simulink model "f16_simulink"  (R2021a)
settings: Solver=VariableStepAuto  StartTime=0.0  StopTime=30  FixedStep=0.01  MaxStep=0.1  RelTol=1e-3
values from neighbouring files (symbols this model uses):
  alpha_vec = -10:5:45    [f16_aeroFM.m]    (also in f16_controlFM.m; f16_simulink_setup.m)
  altitude_vec = 0:10000:50000    [f16_simulink_setup.m]    (also in f16_thrust.m)
  beta_vec10 = -30:10:30    [f16_controlFM.m]    (also in f16_simulink_setup.m)
  beta_vec5 = 0:5:30    [f16_aeroFM.m]    (also in f16_simulink_setup.m)
  Cz_lookup = [.770, .241, -.100, -.416, -.731, -1.053, -1.366, -1.646, -1.917, -2.120, -2.248, -2.229]    [f16_aeroFM.m]    (also in f16_simulink_setup.m)
  damp_table = [-.267, -.110, .308, 1.34, 2.08, 2.91, 2.76, 2.05, 1.50, 1.49, 1.83, 1.21 ... (first row only)    [f16_simulink_setup.m]
  elev_vec = -24:12:24    [f16_aeroFM.m]    (also in f16_simulink_setup.m)
  GAM = mass.Jxx*mass.Jzz - mass.Jxz^2    [f16_dynamics.m]    (also in f16_simulink_setup.m)
  Kp = 0.65    [f16_simulink_DAQ.m]
  Kpi = 0.01    [f16_simulink_DAQ.m]
  Kt = 0.439    [f16_simulink_DAQ.m]
  Mach_vec = linspace(0,1,6)    [f16_simulink_setup.m]    (also in f16_thrust.m)
  OL_cmd = 15    [f16_simulink_DAQ.m]
  pilot_delay = 0.15    [f16_simulink_DAQ.m]
  pitch_limiter = 70    [f16_simulink_DAQ.m]
  pow_vec = [0 50 100]    [f16_simulink_setup.m]    (also in f16_thrust.m)
  power_table = cat(3,throt1',throt2',throt3')    [f16_simulink_setup.m]
  pulse_on = 0    [f16_simulink_DAQ.m]
  r2d = 57.29578    [f16_dynamics.m]    (also in f16_simulink_setup.m = 57.2957795131)
  ratelim_on = 1    [f16_simulink_DAQ.m]
  rho0 = 2.377e-3    (= 0.002377)    [f16_simulink_setup.m]
  thetaref_amp = 20    [f16_simulink_DAQ.m]
  thetaref_per = 4    [f16_simulink_DAQ.m]
  utrim = [smin(1) smin(2) smin(4) smin(5)]'    [f16_DAQ.m]    (also in f16_simulink_DAQ.m)
  wavestart = 5    [f16_simulink_DAQ.m]    (also in f16_simulink_setup.m)
  xcgr = 0.3    [f16_simulink_DAQ.m]
  xPQ = mass.Jxz*(mass.Jxx - mass.Jyy + mass.Jzz)    [f16_dynamics.m]    (also in f16_simulink_setup.m)
  xQR = mass.Jzz*(mass.Jzz-mass.Jyy) + mass.Jxz*2    [f16_dynamics.m]    (also in f16_simulink_setup.m)
  xtrim = x    [f16_DAQ.m]    (also in f16_simulink_DAQ.m)
  yPR = mass.Jzz - mass.Jxx    [f16_dynamics.m]    (also in f16_simulink_setup.m)
  zPQ = (mass.Jxx - mass.Jyy)*mass.Jxx + mass.Jxz^2    [f16_dynamics.m]    (also in f16_simulink_setup.m)
undefined symbols (not defined in the file or in its folder): ctrl, dims, mass
settings Model: Creator=loren  LastModifiedBy=loren

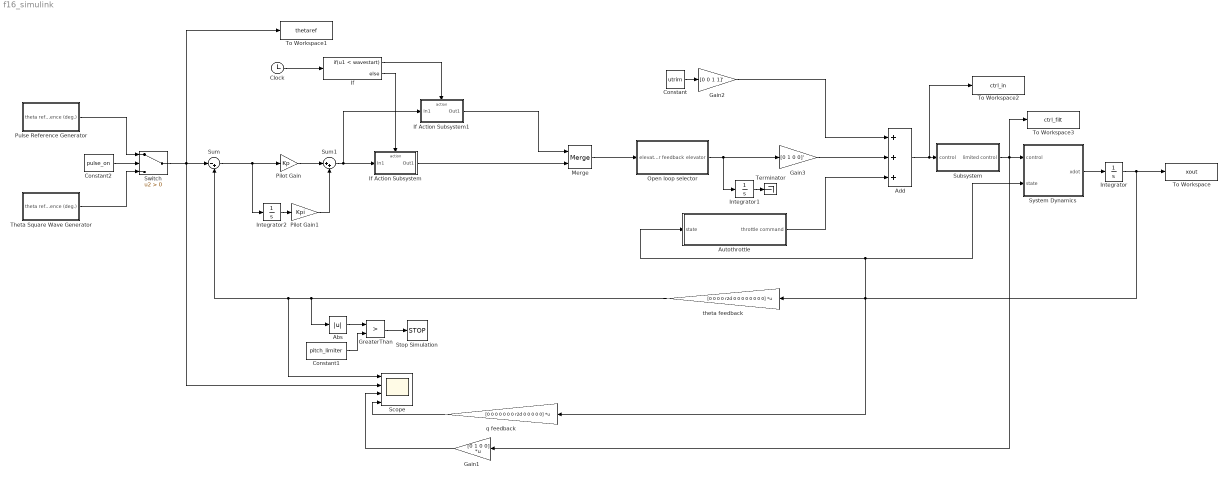
== system f16_simulink ==
  Abs : Abs
  Add : Sum  Inputs=+++
  Autothrottle : Subsystem
  Clock : Clock
  Constant : Constant  Value=utrim
  Constant1 : Constant  Value=pitch_limiter
  Constant2 : Constant  Value=pulse_on
  Gain1 : Gain  Gain=[0 1 0 0]  Multiplication=Matrix(K*u)
  Gain2 : Gain  Gain=[0 0 1 1]'
  Gain3 : Gain  Gain=[0 1 0 0]'
  GreaterThan : RelationalOperator  Operator=>  OutDataTypeStr=boolean  RndMeth=Simplest
  If : If  IfExpression=u1 < wavestart
  If Action Subsystem : Subsystem  TreatAsAtomicUnit=on
  If Action Subsystem1 : Subsystem  TreatAsAtomicUnit=on
  Integrator : Integrator  InitialCondition=xtrim
  Integrator1 : Integrator  InitialCondition=utrim(2)
  Integrator2 : Integrator  InitialCondition=utrim(2)*1000
  Merge : Merge
  Open loop selector : Subsystem
  Pilot Gain : Gain  Gain=Kp
  Pilot Gain1 : Gain  Gain=Kpi
  Pulse Reference Generator : Subsystem
  Scope : Scope  NumInputPorts=4
  Stop Simulation : Stop
  Subsystem : Subsystem
  Sum : Sum  Inputs=|-+
  Sum1 : Sum  Inputs=|++
  Switch : Switch  Criteria=u2 > Threshold
  System Dynamics : Subsystem
  Terminator : Terminator
  Theta Square Wave Generator : Subsystem
  To Workspace : ToWorkspace  VariableName=xout  SampleTime=-1
  To Workspace1 : ToWorkspace  VariableName=thetaref  SampleTime=-1
  To Workspace2 : ToWorkspace  VariableName=ctrl_in  SampleTime=-1
  To Workspace3 : ToWorkspace  VariableName=ctrl_filt  SampleTime=-1
  q feedback : Gain  Gain=[0 0 0 0 0 0 0 r2d 0 0 0 0 0]  Multiplication=Matrix(K*u)
  theta feedback : Gain  Gain=[0 0 0 0 r2d 0 0 0 0 0 0 0 0]  Multiplication=Matrix(K*u)
  wires:
  System Dynamics/1(xdot) -> Integrator/1
  Integrator/1 -> q feedback/1, theta feedback/1, Autothrottle/1(state), System Dynamics/2(state), To Workspace/1
  Switch/1 -> To Workspace1/1, Sum/1, Scope/2
  Sum1/1 -> If Action Subsystem1/1(In1), If Action Subsystem/1(In1)
  Subsystem/1(limited control) -> To Workspace3/1, Gain1/1, System Dynamics/1(control)
  Sum/1 -> Integrator2/1, Pilot Gain/1
  Add/1 -> To Workspace2/1, Subsystem/1(control)
  Constant/1 -> Gain2/1
  Gain2/1 -> Add/1
  Autothrottle/1(throttle command) -> Add/3
  theta feedback/1 -> Abs/1, Sum/2, Scope/1
  Gain1/1 -> Scope/3
  GreaterThan/1 -> Stop Simulation/1
  Abs/1 -> GreaterThan/1
  Constant1/1 -> GreaterThan/2
  Constant2/1 -> Switch/2
  Pulse Reference Generator/1(theta reference (deg.)) -> Switch/1
  Theta Square Wave Generator/1(theta reference (deg.)) -> Switch/3
  q feedback/1 -> Scope/4
  Gain3/1 -> Add/2
  Open loop selector/1(elevator) -> Integrator1/1, Gain3/1
  Integrator1/1 -> Terminator/1
  Integrator2/1 -> Pilot Gain1/1
  Pilot Gain1/1 -> Sum1/2
  Merge/1 -> Open loop selector/1(elevator feedback)
  Pilot Gain/1 -> Sum1/1
  Clock/1 -> If/1
  If Action Subsystem1/1(Out1) -> Merge/1
  If/2 -> If Action Subsystem/Action
  If/1 -> If Action Subsystem1/Action
  If Action Subsystem/1(Out1) -> Merge/2

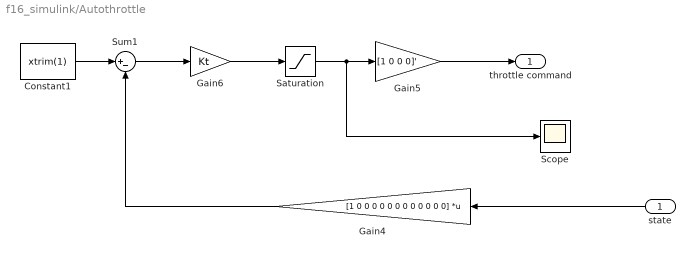
== system f16_simulink/Autothrottle ==
  state : Inport
  Constant1 : Constant  Value=xtrim(1)
  Gain4 : Gain  Gain=[1 0 0 0 0 0 0 0 0 0 0 0 0]  Multiplication=Matrix(K*u)
  Gain5 : Gain  Gain=[1 0 0 0]'
  Gain6 : Gain  Gain=Kt
  Saturation : Saturate  UpperLimit=1  LowerLimit=0.1
  Scope : Scope
  Sum1 : Sum  Inputs=|+-
  throttle command : Outport
  wires:
  Saturation/1 -> Scope/1, Gain5/1
  Sum1/1 -> Gain6/1
  Gain4/1 -> Sum1/2
  Gain5/1 -> throttle command/1
  state/1 -> Gain4/1
  Constant1/1 -> Sum1/1
  Gain6/1 -> Saturation/1

== system f16_simulink/If Action Subsystem ==
  In1 : Inport
  Action Port : ActionPort  ActionPortLabel=else
  Pilot Delay1 : TransportDelay  DelayTime=pilot_delay
  Out1 : Outport
  wires:
  In1/1 -> Pilot Delay1/1
  Pilot Delay1/1 -> Out1/1

== system f16_simulink/If Action Subsystem1 ==
  In1 : Inport
  Action Port : ActionPort  ActionPortLabel=if(u1 < wavestart)
  Out1 : Outport
  wires:
  In1/1 -> Out1/1

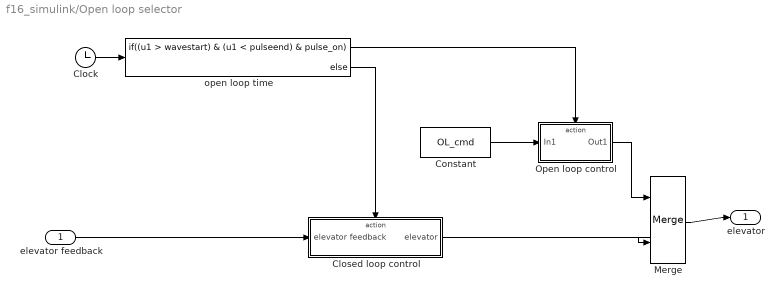
== system f16_simulink/Open loop selector ==
  elevator feedback : Inport
  Clock : Clock
  Closed loop control : Subsystem  TreatAsAtomicUnit=on
  Constant : Constant  Value=OL_cmd
  Merge : Merge
  Open loop control : Subsystem  TreatAsAtomicUnit=on
  open loop time : If  IfExpression=(u1 > wavestart) & (u1 < pulseend) & pulse_on
  elevator : Outport
  wires:
  Clock/1 -> open loop time/1
  Merge/1 -> elevator/1
  elevator feedback/1 -> Closed loop control/1(elevator feedback)
  open loop time/2 -> Closed loop control/Action
  Closed loop control/1(elevator) -> Merge/2
  Open loop control/1(Out1) -> Merge/1
  open loop time/1 -> Open loop control/Action
  Constant/1 -> Open loop control/1(In1)

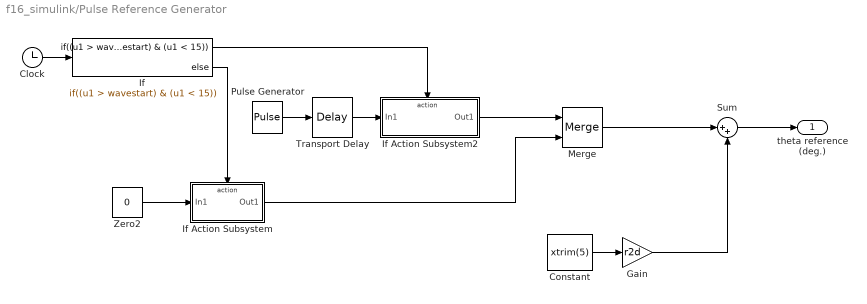
== system f16_simulink/Pulse Reference Generator ==
  Clock : Clock
  Constant : Constant  Value=xtrim(5)
  Gain : Gain  Gain=r2d
  If : If  IfExpression=(u1 > wavestart) & (u1 < 15)
  If Action Subsystem : Subsystem  TreatAsAtomicUnit=on
  If Action Subsystem2 : Subsystem  TreatAsAtomicUnit=on
  Merge : Merge
  Pulse Generator : DiscretePulseGenerator  PulseType=Time based  Amplitude=0  Period=20  PulseWidth=50
  Sum : Sum  Inputs=|++
  Transport Delay : TransportDelay  DelayTime=wavestart
  Zero2 : Constant  Value=0  OutDataTypeStr=Inherit: Inherit via back propagation
  theta reference (deg.) : Outport
  wires:
  Sum/1 -> theta reference (deg.)/1
  Pulse Generator/1 -> Transport Delay/1
  Gain/1 -> Sum/2
  Constant/1 -> Gain/1
  Merge/1 -> Sum/1
  If Action Subsystem2/1(Out1) -> Merge/1
  If/1 -> If Action Subsystem2/Action
  Clock/1 -> If/1
  If/2 -> If Action Subsystem/Action
  Transport Delay/1 -> If Action Subsystem2/1(In1)
  If Action Subsystem/1(Out1) -> Merge/2
  Zero2/1 -> If Action Subsystem/1(In1)

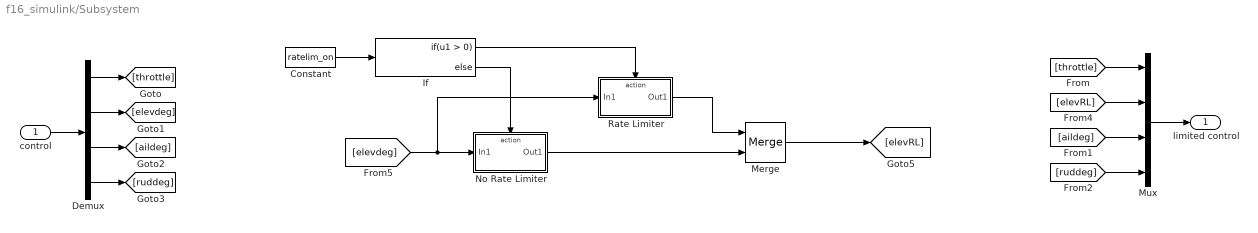
== system f16_simulink/Subsystem ==
  control : Inport
  Constant : Constant  Value=ratelim_on
  Demux : Demux
  If : If
  Merge : Merge
  Mux : Mux
  No Rate Limiter : Subsystem  TreatAsAtomicUnit=on
  Rate Limiter : Subsystem  TreatAsAtomicUnit=on
  limited control : Outport
  wires:
  Mux/1 -> limited control/1
  control/1 -> Demux/1
  Demux/1 -> [throttle]
  Demux/4 -> [ruddeg]
  Demux/3 -> [aildeg]
  Demux/2 -> [elevdeg]
  [throttle] -> Mux/1
  [aildeg] -> Mux/3
  [ruddeg] -> Mux/4
  [elevRL] -> Mux/2
  Constant/1 -> If/1
  If/2 -> No Rate Limiter/Action
  If/1 -> Rate Limiter/Action
  [elevdeg] -> Rate Limiter/1(In1), No Rate Limiter/1(In1)
  Rate Limiter/1(Out1) -> Merge/1
  Merge/1 -> [elevRL]
  No Rate Limiter/1(Out1) -> Merge/2

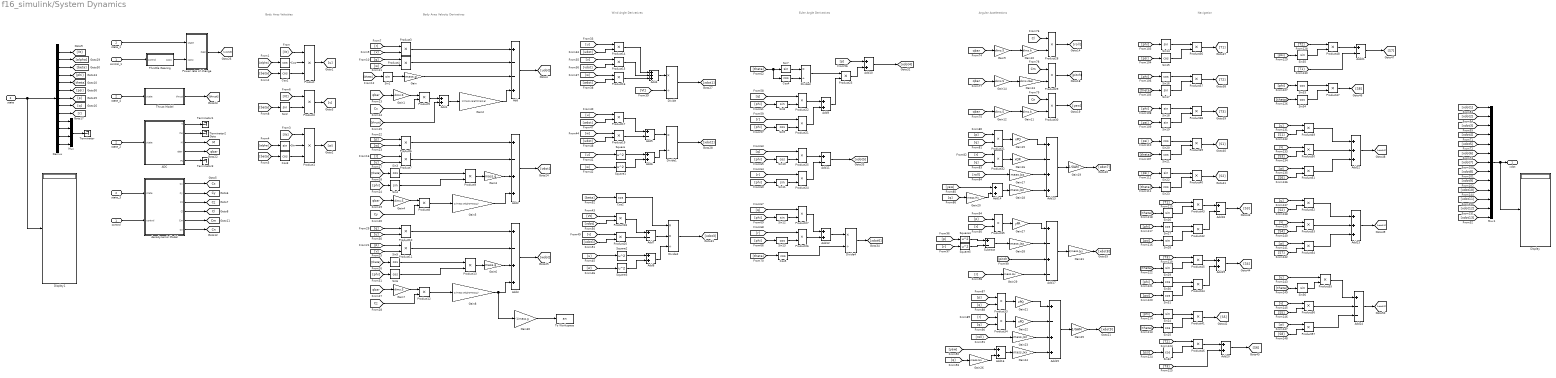
== system f16_simulink/System Dynamics ==
  note: Body Axes Velocities
  note: Body Axes Velocity Derivatives
  note: Wind Angle Derivatives
  note: Euler Angle Derivatives
  note: Angular Accelerations
  note: Navigation
  control : Inport
  state : Inport  Port=2
  ADC : Subsystem
  Add : Sum  Inputs=+--+
  Add{1,6,8..10,12,14,16,19..20} (10 alike) : Sum
  Add{5,7,11,18,21} (5 alike) : Sum  Inputs=+-
  Add{2..3,13,15} (4 alike) : Sum  Inputs=+-++
  Add17 : Sum  Inputs=+-+-
  Add22 : Sum  Inputs=+++
  Add23 : Sum  Inputs=+++
  Add24 : Sum  Inputs=+--
  Add4 : Sum  Inputs=+++
  Aerodynamic Model : Subsystem
  Cos{,1..5} (6 alike) : Trigonometry  Operator=cos
  Demux : Demux  Outputs=13
  Display : Display
  Display1 : Display
  Divide{,1,3..4} (4 alike) : Product  Inputs=*/
  Divide2 : Product  Inputs=**/
  Gain : Gain  Gain=mass.g
  Gain{1,4,7,9,12,14} (6 alike) : Gain  Gain=dims.S
  Gain10 : Gain  Gain=dims.b
  Gain11 : Gain  Gain=dims.b
  Gain13 : Gain  Gain=dims.cbar
  Gain15 : Gain  Gain=xPQ
  Gain16 : Gain  Gain=xQR
  Gain17 : Gain  Gain=mass.Jzz
  Gain18 : Gain  Gain=mass.Jxz
  Gain19 : Gain  Gain=1/GAM
  Gain2 : Gain  Gain=1/(mass.weight/mass.g)
  Gain20 : Gain  Gain=mass.Hx
  Gain21 : Gain  Gain=zPQ
  Gain22 : Gain  Gain=xPQ
  Gain23 : Gain  Gain=mass.Jxz
  Gain24 : Gain  Gain=mass.Jxx
  Gain25 : Gain  Gain=1/GAM
  Gain26 : Gain  Gain=mass.Hx
  Gain27 : Gain  Gain=yPR
  Gain28 : Gain  Gain=mass.Jxz
  Gain29 : Gain  Gain=mass.Hx
  Gain3 : Gain  Gain=mass.g
  Gain30 : Gain  Gain=-1/mass.g
  Gain31 : Gain  Gain=1/mass.Jyy
  Gain5 : Gain  Gain=1/(mass.weight/mass.g)
  Gain6 : Gain  Gain=mass.g
  Gain8 : Gain  Gain=1/(mass.weight/mass.g)
  Mux : Mux
  Mux1 : Mux  Inputs=13
  Power rate of change : Subsystem
  Product : Product  Inputs=3
  Product1 : Product  Inputs=3
  Product{2..57} (56 alike) : Product
  Sin{,1..2,4,7..8,11..12,14,17..19,22,24,26,28..29,35..36} (19 alike) : Trigonometry
  Sin{3,5..6,9..10,13,15..16,20..21,23,25,27,30..34} (18 alike) : Trigonometry  Operator=cos
  Square{,1..5} (6 alike) : Math  Operator=square  SaturateOnIntegerOverflow=on
  Subtract : Sum  Inputs=+-
  Terminator{,1..3} (4 alike) : Terminator
  Throttle Gearing : Subsystem
  Thrust Model : Subsystem
  To Workspace : ToWorkspace  VariableName=an  SampleTime=-1
  control_1 : InportShadow
  state_{1..4} (4 alike) : InportShadow  Port=2
  xdot : Outport
  tag scope: Cl=global, Cm=global, Cn=global, Cx=global, Cy=global, Cz=global, M=global, qbar=global
  wires:
  state_3/1 -> Aerodynamic Model/1(state)
  Add/1 -> [udot]
  [v] -> Product3/2
  [qbar] -> Gain1/1
  ADC/4(qbar) -> [qbar]
  Aerodynamic Model/1(Cx) -> [Cx]
  Thrust Model/1(thrust) -> [thrust]
  Gain/1 -> Add/3
  Mux1/1 -> Display/1, xdot/1
  Throttle Gearing/1(cpow) -> Power rate of change/2(cpow)
  [Vt] -> Product2/1
  [beta] -> Cos1/1
  Add1/1 -> Gain2/1
  ADC/3(M) -> [M]
  state/1 -> Display1/1, Demux/1
  [theta] -> Sin1/1
  Demux/1 -> [Vt]
  Aerodynamic Model/4(Cl) -> [Cl]
  control/1 -> Aerodynamic Model/2(control)
  Demux/13 -> Mux/4
  Demux/5 -> [theta]
  Demux/4 -> [phi]
  Product1/1 -> [w]
  Product2/1 -> [v]
  [Cx] -> Product5/2
  control_1/1 -> Throttle Gearing/1(control)
  state_2/1 -> ADC/1(state)
  Aerodynamic Model/3(Cz) -> [Cz]
  Gain1/1 -> Product5/1
  state_1/1 -> Power rate of change/1(state)
  [alpha] -> Cos/1
  Demux/11 -> Mux/2
  ADC/2(rho) -> Terminator2/1
  Demux/12 -> Mux/3
  Demux/9 -> [r]
  state_4/1 -> Thrust Model/1(state)
  Aerodynamic Model/5(Cm) -> [Cm]
  Aerodynamic Model/6(Cn) -> [Cn]
  [q] -> Product4/1
  [beta] -> Cos3/1
  Demux/7 -> [p]
  Demux/3 -> [beta]
  Aerodynamic Model/2(Cy) -> [Cy]
  Sin2/1 -> Product2/2
  [beta] -> Sin2/1
  Demux/2 -> [alpha]
  ADC/5(Ps) -> Terminator3/1
  Sin1/1 -> Gain/1
  Demux/8 -> [q]
  Mux/1 -> Terminator/1
  Product5/1 -> Add1/1
  Demux/6 -> [psi]
  Demux/10 -> Mux/1
  [Vt] -> Product1/1
  Sin/1 -> Product1/2
  Product3/1 -> Add/1
  [thrust] -> Add1/2
  Product/1 -> [u]
  Cos3/1 -> Product1/3
  [alpha] -> Sin/1
  Cos/1 -> Product/2
  [r] -> Product3/1
  Product4/1 -> Add/2
  [Vt] -> Product/1
  [w] -> Product4/2
  Cos1/1 -> Product/3
  Gain2/1 -> Add/4
  ADC/1(T) -> Terminator1/1
  Power rate of change/1(Pdot) -> [xdot13]
  Gain4/1 -> Product8/1
  [Cy] -> Product8/2
  [theta] -> Sin3/1
  Product8/1 -> Gain5/1
  [qbar] -> Gain4/1
  Sin3/1 -> Product9/1
  [w] -> Product6/2
  Add2/1 -> [vdot]
  Gain5/1 -> Add2/4
  [u] -> Product7/2
  Product7/1 -> Add2/2
  [p] -> Product6/1
  [r] -> Product7/1
  Product6/1 -> Add2/1
  Product9/1 -> Gain3/1
  [phi] -> Sin4/1
  Sin4/1 -> Product9/2
  Gain3/1 -> Add2/3
  [phi] -> Sin6/1
  [p] -> Product11/1
  [q] -> Product10/1
  Product11/1 -> Add3/2
  [Cz] -> Product12/2
  [u] -> Product10/2
  [qbar] -> Gain7/1
  [theta] -> Sin5/1
  Gain7/1 -> Product12/1
  Product12/1 -> Gain8/1
  Product10/1 -> Add3/1
  Add3/1 -> [wdot]
  Gain6/1 -> Add3/3
  Sin6/1 -> Product13/2
  Product13/1 -> Gain6/1
  Gain8/1 -> Gain30/1, Add3/4
  Sin5/1 -> Product13/1
  [v] -> Product11/2
  [xdot13] -> Mux1/13
  [u] -> Product14/1
  [udot] -> Product14/2
  [v] -> Product15/1
  [w] -> Product16/1
  [vdot] -> Product15/2
  [wdot] -> Product16/2
  Product15/1 -> Add4/2
  Product14/1 -> Add4/1
  Product16/1 -> Add4/3
  Add4/1 -> Divide/1
  [Vt] -> Divide/2
  Divide/1 -> [xdot1]
  [udot] -> Product19/2
  [wdot] -> Product17/2
  [u] -> Product17/1
  [w] -> Product19/1
  Product17/1 -> Add5/1
  Add5/1 -> Divide1/1
  Add6/1 -> Divide1/2
  Divide1/1 -> [xdot2]
  Product19/1 -> Add5/2
  [w] -> Square1/1
  Square1/1 -> Add6/2
  Square/1 -> Add6/1
  [u] -> Square/1
  [w] -> Square3/1
  [vdot] -> Product18/2
  Add8/1 -> Divide2/3
  Product20/1 -> Add7/2
  [u] -> Square2/1
  [xdot1] -> Product20/2
  Divide2/1 -> [xdot3]
  Square3/1 -> Add8/2
  Add7/1 -> Divide2/2
  Product18/1 -> Add7/1
  [Vt] -> Product18/1
  Square2/1 -> Add8/1
  [v] -> Product20/1
  Cos2/1 -> Divide2/1
  [beta] -> Cos2/1
  [xdot3] -> Mux1/3
  [xdot2] -> Mux1/2
  [xdot1] -> Mux1/1
  [theta] -> Cos4/1, Sin7/1
  Sin7/1 -> Divide3/1
  Cos4/1 -> Divide3/2
  [phi] -> Sin8/1
  [phi] -> Sin9/1
  Sin9/1 -> Product21/2
  Sin8/1 -> Product22/2
  [r] -> Product21/1
  [q] -> Product22/1
  Product22/1 -> Add9/1
  Product21/1 -> Add9/2
  Divide3/1 -> Product23/1
  Add9/1 -> Product23/2
  [p] -> Add10/1
  Product23/1 -> Add10/2
  Add10/1 -> [xdot4]
  Product24/1 -> Add11/2
  [r] -> Product24/1
  [phi] -> Sin11/1
  Sin10/1 -> Product25/2
  [q] -> Product25/1
  [phi] -> Sin10/1
  Product25/1 -> Add11/1
  Sin11/1 -> Product24/2
  Product26/1 -> Add12/2
  [r] -> Product26/1
  [phi] -> Sin13/1
  Sin12/1 -> Product27/2
  [q] -> Product27/1
  [phi] -> Sin12/1
  Product27/1 -> Add12/1
  Sin13/1 -> Product26/2
  Add12/1 -> Divide4/1
  [theta] -> Cos5/1
  Cos5/1 -> Divide4/2
  Add11/1 -> [xdot5]
  Divide4/1 -> [xdot6]
  [xdot4] -> Mux1/4
  [xdot5] -> Mux1/5
  [xdot6] -> Mux1/6
  [qbar] -> Gain9/1
  Gain9/1 -> Gain10/1
  Gain10/1 -> Product28/2
  [Cl] -> Product28/1
  Product28/1 -> [roll]
  Gain13/1 -> Product29/2
  Product29/1 -> [pitch]
  [Cm] -> Product29/1
  [qbar] -> Gain14/1
  Gain14/1 -> Gain13/1
  Gain11/1 -> Product30/2
  Product30/1 -> [yaw]
  [Cn] -> Product30/1
  [qbar] -> Gain12/1
  Gain12/1 -> Gain11/1
  [p] -> Product31/1
  [q] -> Product31/2
  Product31/1 -> Gain15/1
  Gain15/1 -> Add13/1
  Product32/1 -> Gain16/1
  [r] -> Product32/1
  [q] -> Product32/2
  Gain16/1 -> Add13/2
  [roll] -> Gain17/1
  Gain17/1 -> Add13/3
  Gain18/1 -> Add13/4
  Add13/1 -> Gain19/1
  Gain19/1 -> [xdot7]
  Add14/1 -> Gain18/1
  [yaw] -> Add14/1
  [q] -> Gain20/1
  Gain20/1 -> Add14/2
  Gain26/1 -> Add16/2
  [q] -> Gain26/1
  [yaw] -> Add16/1
  Add16/1 -> Gain24/1
  Gain25/1 -> [xdot9]
  Add15/1 -> Gain25/1
  Gain24/1 -> Add15/4
  Gain23/1 -> Add15/3
  [roll] -> Gain23/1
  Gain22/1 -> Add15/2
  [q] -> Product34/2
  [r] -> Product34/1
  Product34/1 -> Gain22/1
  Gain21/1 -> Add15/1
  Product33/1 -> Gain21/1
  [q] -> Product33/2
  [p] -> Product33/1
  [r] -> Product35/2
  Gain27/1 -> Add17/1
  Add17/1 -> Gain31/1
  [p] -> Product35/1
  Gain31/1 -> [xdot8]
  Product35/1 -> Gain27/1
  Gain28/1 -> Add17/2
  Subtract/1 -> Gain28/1
  [p] -> Square4/1
  [r] -> Square5/1
  Square5/1 -> Subtract/2
  Square4/1 -> Subtract/1
  [r] -> Gain29/1
  [pitch] -> Add17/3
  [xdot7] -> Mux1/7
  [xdot8] -> Mux1/8
  [xdot9] -> Mux1/9
  [phi] -> Sin14/1
  [psi] -> Sin15/1
  Sin14/1 -> Product36/1
  Sin15/1 -> Product36/2
  Product36/1 -> [T1]
  Product37/1 -> [T2]
  [phi] -> Sin16/1
  Sin16/1 -> Product37/1
  Sin17/1 -> Product37/2
  [theta] -> Sin17/1
  Product38/1 -> [T3]
  Sin19/1 -> Product38/2
  Sin18/1 -> Product38/1
  [psi] -> Sin19/1
  [phi] -> Sin18/1
  [theta] -> Sin21/1
  Sin21/1 -> Product39/2
  Sin20/1 -> Product39/1
  [psi] -> Sin20/1
  Product39/1 -> [S1]
  Product40/1 -> [S2]
  [psi] -> Sin22/1
  Sin22/1 -> Product40/1
  Sin23/1 -> Product40/2
  [theta] -> Sin23/1
  [theta] -> Sin25/1
  Sin25/1 -> Product41/2
  Sin24/1 -> Product41/1
  [phi] -> Sin24/1
  Product41/1 -> [S5]
  [psi] -> Sin28/1
  Sin28/1 -> Product42/2
  Sin27/1 -> Product42/1
  [phi] -> Sin27/1
  [T1] -> Product43/1
  Sin26/1 -> Product43/2
  [theta] -> Sin26/1
  Product43/1 -> Add18/1
  Product42/1 -> Add18/2
  Add18/1 -> [S3]
  Add19/1 -> [S4]
  Product44/1 -> Add19/2
  Product45/1 -> Add19/1
  [theta] -> Sin29/1
  Sin29/1 -> Product45/2
  [T3] -> Product45/1
  [phi] -> Sin30/1
  Sin30/1 -> Product44/1
  Sin31/1 -> Product44/2
  [psi] -> Sin31/1
  [psi] -> Sin32/1
  Sin32/1 -> Product46/2
  [T2] -> Product46/1
  Product46/1 -> Add20/1
  [T3] -> Add20/2
  Add20/1 -> [S6]
  Product47/1 -> [S8]
  [phi] -> Sin33/1
  Sin33/1 -> Product47/1
  Sin34/1 -> Product47/2
  [theta] -> Sin34/1
  Add21/1 -> [S7]
  [T1] -> Add21/2
  Product48/1 -> Add21/1
  [T2] -> Product48/1
  Sin35/1 -> Product48/2
  [psi] -> Sin35/1
  [u] -> Product49/1
  [S1] -> Product49/2
  Product49/1 -> Add22/1
  [S3] -> Product50/2
  [v] -> Product50/1
  Product50/1 -> Add22/2
  [w] -> Product51/1
  [S6] -> Product51/2
  Product51/1 -> Add22/3
  Add22/1 -> [xdot10]
  Add23/1 -> [xdot11]
  Product54/1 -> Add23/3
  [S7] -> Product54/2
  [w] -> Product54/1
  Product53/1 -> Add23/2
  [v] -> Product53/1
  [S4] -> Product53/2
  Product52/1 -> Add23/1
  [S2] -> Product52/2
  [u] -> Product52/1
  [u] -> Product55/1
  Sin36/1 -> Product55/2
  Product55/1 -> Add24/1
  [S5] -> Product56/2
  [v] -> Product56/1
  Product56/1 -> Add24/2
  [w] -> Product57/1
  [S8] -> Product57/2
  Product57/1 -> Add24/3
  Add24/1 -> [xdot12]
  [theta] -> Sin36/1
  [xdot12] -> Mux1/12
  [xdot11] -> Mux1/11
  [xdot10] -> Mux1/10
  Gain29/1 -> Add17/4
  Gain30/1 -> To Workspace/1

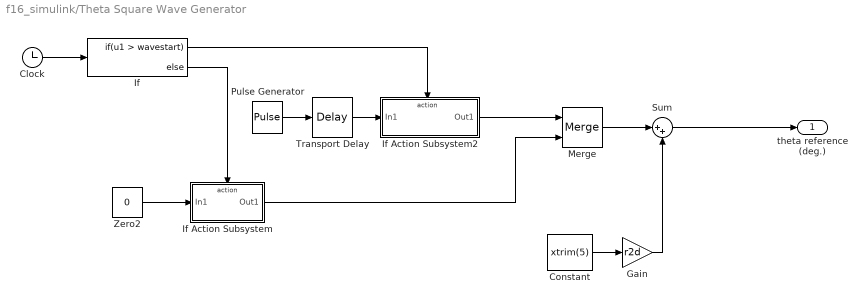
== system f16_simulink/Theta Square Wave Generator ==
  Clock : Clock
  Constant : Constant  Value=xtrim(5)
  Gain : Gain  Gain=r2d
  If : If  IfExpression=u1 > wavestart
  If Action Subsystem : Subsystem  TreatAsAtomicUnit=on
  If Action Subsystem2 : Subsystem  TreatAsAtomicUnit=on
  Merge : Merge
  Pulse Generator : DiscretePulseGenerator  PulseType=Time based  Amplitude=2*thetaref_amp  Period=thetaref_per  PulseWidth=50
  Sum : Sum  Inputs=|++
  Transport Delay : TransportDelay  DelayTime=wavestart
  Zero2 : Constant  Value=0  OutDataTypeStr=Inherit: Inherit via back propagation
  theta reference (deg.) : Outport
  wires:
  Zero2/1 -> If Action Subsystem/1(In1)
  If Action Subsystem/1(Out1) -> Merge/2
  Transport Delay/1 -> If Action Subsystem2/1(In1)
  If/2 -> If Action Subsystem/Action
  Clock/1 -> If/1
  If/1 -> If Action Subsystem2/Action
  If Action Subsystem2/1(Out1) -> Merge/1
  Merge/1 -> Sum/1
  Constant/1 -> Gain/1
  Gain/1 -> Sum/2
  Pulse Generator/1 -> Transport Delay/1
  Sum/1 -> theta reference (deg.)/1

== system f16_simulink/Open loop selector/Closed loop control ==
  elevator feedback : Inport
  Action Port : ActionPort  ActionPortLabel=else
  elevator : Outport
  wires:
  elevator feedback/1 -> elevator/1

== system f16_simulink/Open loop selector/Open loop control ==
  In1 : Inport
  Action Port : ActionPort  ActionPortLabel=if((u1 > wavestart) & (u1 < pulseend) & pulse_on)
  Out1 : Outport
  wires:
  In1/1 -> Out1/1

== system f16_simulink/Pulse Reference Generator/If Action Subsystem ==
  In1 : Inport
  Action Port : ActionPort  ActionPortLabel=else
  Out1 : Outport
  wires:
  In1/1 -> Out1/1

== system f16_simulink/Pulse Reference Generator/If Action Subsystem2 ==
  In1 : Inport
  Action Port : ActionPort  ActionPortLabel=if((u1 > wavestart) & (u1 < 15))
  Out1 : Outport
  wires:
  In1/1 -> Out1/1

== system f16_simulink/Subsystem/No Rate Limiter ==
  In1 : Inport
  Action Port : ActionPort  ActionPortLabel=else
  Elevator Saturation : Saturate  UpperLimit=ctrl.elev.satlim  LowerLimit=-ctrl.elev.satlim
  Out1 : Outport
  wires:
  In1/1 -> Elevator Saturation/1
  Elevator Saturation/1 -> Out1/1

== system f16_simulink/Subsystem/Rate Limiter ==
  In1 : Inport
  Action Port : ActionPort  ActionPortLabel=if(u1 > 0)
  Elevator Saturation : Saturate  UpperLimit=ctrl.elev.satlim  LowerLimit=-ctrl.elev.satlim
  Elevator Rate Limiter : RateLimiter  RisingSlewLimit=ctrl.elev.ratelim  FallingSlewLimit=-ctrl.elev.ratelim
  Scope : Scope  NumInputPorts=2
  Out1 : Outport
  wires:
  Elevator Saturation/1 -> Out1/1
  Elevator Rate Limiter/1 -> Scope/2, Elevator Saturation/1
  In1/1 -> Scope/1, Elevator Rate Limiter/1

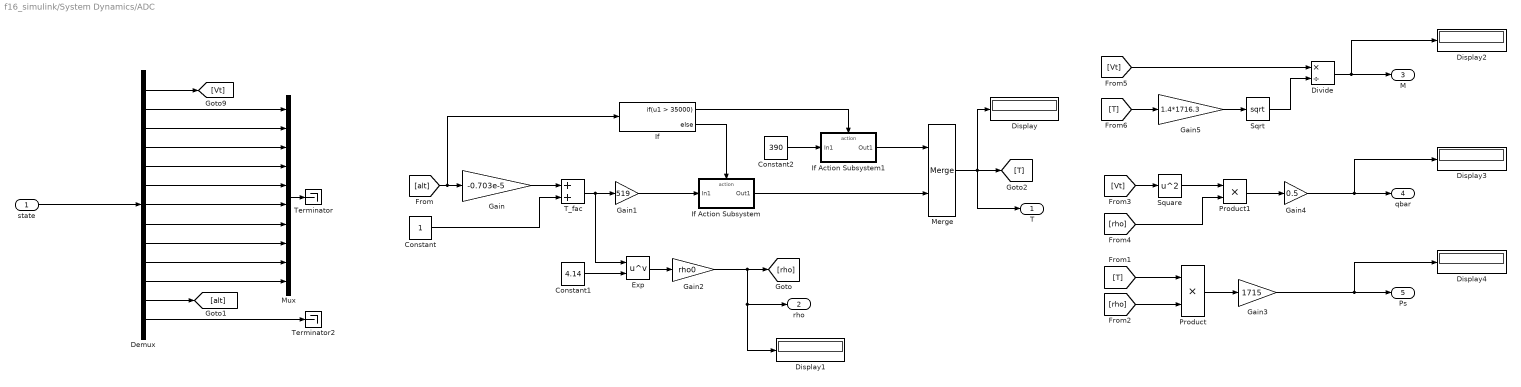
== system f16_simulink/System Dynamics/ADC ==
  state : Inport
  Constant : Constant
  Constant1 : Constant  Value=4.14
  Constant2 : Constant  Value=390
  Demux : Demux  Outputs=13
  Display{,1..4} (5 alike) : Display
  Divide : Product  Inputs=*/
  Exp : Math  Operator=pow  SaturateOnIntegerOverflow=on
  Gain : Gain  Gain=-0.703e-5
  Gain1 : Gain  Gain=519
  Gain2 : Gain  Gain=rho0
  Gain3 : Gain  Gain=1715
  Gain4 : Gain  Gain=0.5
  Gain5 : Gain  Gain=1.4*1716.3
  If : If  IfExpression=u1 > 35000
  If Action Subsystem : Subsystem  TreatAsAtomicUnit=on
  If Action Subsystem1 : Subsystem  TreatAsAtomicUnit=on
  Merge : Merge
  Mux : Mux  Inputs=10
  Product : Product
  Product1 : Product
  Sqrt : Sqrt  SaturateOnIntegerOverflow=on
  Square : Math  Operator=square  SaturateOnIntegerOverflow=on
  T_fac : Sum
  Terminator : Terminator
  Terminator2 : Terminator
  T : Outport
  rho : Outport  Port=2
  M : Outport  Port=3
  qbar : Outport  Port=4
  Ps : Outport  Port=5
  wires:
  Gain1/1 -> If Action Subsystem/1(In1)
  Demux/3 -> Mux/2
  T_fac/1 -> Exp/1, Gain1/1
  Product/1 -> Gain3/1
  Demux/10 -> Mux/9
  Constant2/1 -> If Action Subsystem1/1(In1)
  Demux/13 -> Terminator2/1
  Demux/4 -> Mux/3
  Gain4/1 -> qbar/1, Display3/1
  If Action Subsystem/1(Out1) -> Merge/2
  Constant/1 -> T_fac/2
  Demux/2 -> Mux/1
  Gain3/1 -> Ps/1, Display4/1
  Constant1/1 -> Exp/2
  Merge/1 -> T/1, Display/1, [T]
  Gain/1 -> T_fac/1
  [T] -> Product/1
  Sqrt/1 -> Divide/2
  [rho] -> Product1/2
  [T] -> Gain5/1
  Square/1 -> Product1/1
  [alt] -> If/1, Gain/1
  Demux/9 -> Mux/8
  [rho] -> Product/2
  If Action Subsystem1/1(Out1) -> Merge/1
  Divide/1 -> M/1, Display2/1
  Demux/12 -> [alt]
  Gain2/1 -> rho/1, Display1/1, [rho]
  Demux/6 -> Mux/5
  Demux/1 -> [Vt]
  Exp/1 -> Gain2/1
  Gain5/1 -> Sqrt/1
  [Vt] -> Square/1
  [Vt] -> Divide/1
  If/2 -> If Action Subsystem/Action
  Product1/1 -> Gain4/1
  Mux/1 -> Terminator/1
  Demux/11 -> Mux/10
  Demux/5 -> Mux/4
  Demux/7 -> Mux/6
  Demux/8 -> Mux/7
  If/1 -> If Action Subsystem1/Action
  state/1 -> Demux/1

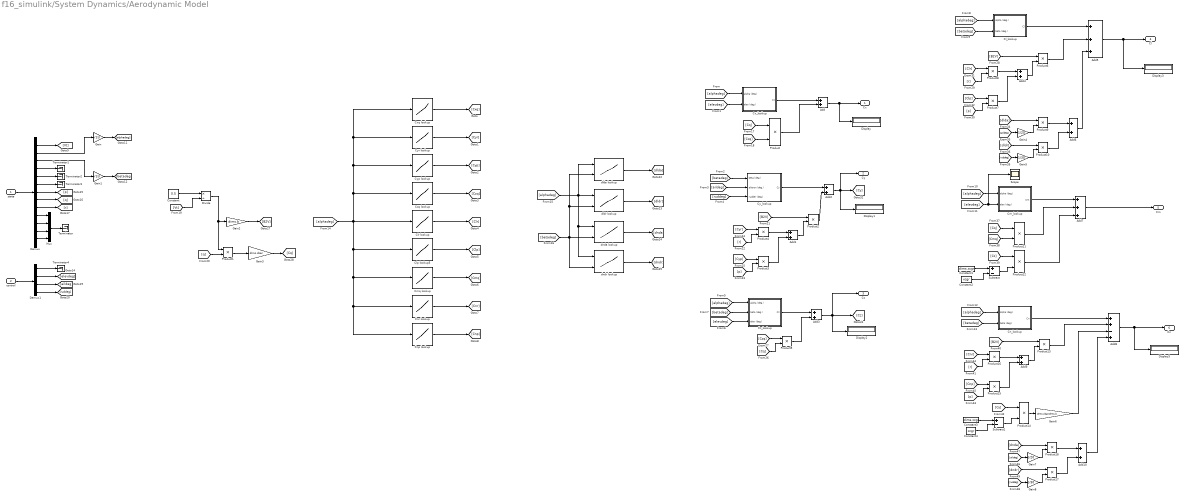
== system f16_simulink/System Dynamics/Aerodynamic Model ==
  state : Inport
  control : Inport  Port=2
  Add{,1..4,6,9..10} (8 alike) : Sum
  Add5 : Sum  Inputs=+++
  Add7 : Sum  Inputs=+++
  Add8 : Sum  Inputs=++-+
  Cl_lookup : Subsystem
  Clp lookup5 : Lookup_n-D  NumberOfTableDimensions=1  BreakpointsForDimension1=alpha_vec  Table=damp_table(6,:)  InternalRulePriority=Speed  RndMeth=Simplest  InputSameDT=on
  Clr lookup : Lookup_n-D  NumberOfTableDimensions=1  BreakpointsForDimension1=alpha_vec  Table=damp_table(5,:)  InternalRulePriority=Speed  RndMeth=Simplest  InputSameDT=on
  Cm_lookup : Subsystem
  Cmq lookup : Lookup_n-D  NumberOfTableDimensions=1  BreakpointsForDimension1=alpha_vec  Table=damp_table(7,:)  InternalRulePriority=Speed  RndMeth=Simplest  InputSameDT=on
  Cn_lookup : Subsystem
  Cnp lookup : Lookup_n-D  NumberOfTableDimensions=1  BreakpointsForDimension1=alpha_vec  Table=damp_table(9,:)  InternalRulePriority=Speed  RndMeth=Simplest  InputSameDT=on
  Cnr lookup : Lookup_n-D  NumberOfTableDimensions=1  BreakpointsForDimension1=alpha_vec  Table=damp_table(8,:)  InternalRulePriority=Speed  RndMeth=Simplest  InputSameDT=on
  Constant : Constant  Value=0.5
  Constant1 : Constant  Value=dims.xcgr
  Constant2 : Constant  Value=xcgr
  Constant3 : Constant  Value=dims.xcgr
  Constant4 : Constant  Value=xcgr
  Cx_lookup : Subsystem
  Cxq lookup : Lookup_n-D  NumberOfTableDimensions=1  BreakpointsForDimension1=alpha_vec  Table=damp_table(1,:)  InternalRulePriority=Speed  RndMeth=Simplest  InputSameDT=on
  Cy_lookup : Subsystem
  Cyp lookup : Lookup_n-D  NumberOfTableDimensions=1  BreakpointsForDimension1=alpha_vec  Table=damp_table(3,:)  InternalRulePriority=Speed  RndMeth=Simplest  InputSameDT=on
  Cyr lookup : Lookup_n-D  NumberOfTableDimensions=1  BreakpointsForDimension1=alpha_vec  Table=damp_table(2,:)  ExtrapMethod=Clip  InternalRulePriority=Speed  RndMeth=Simplest  InputSameDT=on
  Cz_lookup : Subsystem
  Czq lookup : Lookup_n-D  NumberOfTableDimensions=1  BreakpointsForDimension1=alpha_vec  Table=damp_table(4,:)  InternalRulePriority=Speed  RndMeth=Simplest  InputSameDT=on
  Demux : Demux  Outputs=13
  Demux1 : Demux
  Display{,1..3,5} (5 alike) : Display
  Divide : Product  Inputs=*/
  Gain : Gain  Gain=r2d
  Gain1 : Gain  Gain=r2d
  Gain2 : Gain  Gain=dims.b
  Gain3 : Gain  Gain=dims.cbar
  Gain4 : Gain  Gain=1/20
  Gain5 : Gain  Gain=1/30
  Gain6 : Gain  Gain=dims.cbar/dims.b
  Gain7 : Gain  Gain=1/20
  Gain8 : Gain  Gain=1/30
  Mux : Mux
  Product{,1..18} (19 alike) : Product
  Scope : Scope
  Subtract : Sum  Inputs=+-
  Subtract1 : Sum  Inputs=+-
  Terminator{,1..4} (5 alike) : Terminator
  dlda lookup : Lookup_n-D  BreakpointsForDimension1=alpha_vec  BreakpointsForDimension2=beta_vec10  BreakpointsForDimension3=[5, 7]  Table=dlda_lookup'  InternalRulePriority=Speed  RndMeth=Simplest  InputSameDT=on
      settings: InputPortMap=u0,u1
  dldr lookup : Lookup_n-D  BreakpointsForDimension1=alpha_vec  BreakpointsForDimension2=beta_vec10  BreakpointsForDimension3=[5, 7]  Table=dldr_lookup'  InternalRulePriority=Speed  RndMeth=Simplest  InputSameDT=on
      settings: InputPortMap=u0,u1
  dnda lookup : Lookup_n-D  BreakpointsForDimension1=alpha_vec  BreakpointsForDimension2=beta_vec10  BreakpointsForDimension3=[5, 7]  Table=dnda_lookup'  InternalRulePriority=Speed  RndMeth=Simplest  InputSameDT=on
      settings: InputPortMap=u0,u1
  dndr lookup : Lookup_n-D  BreakpointsForDimension1=alpha_vec  BreakpointsForDimension2=beta_vec10  BreakpointsForDimension3=[5, 7]  Table=dndr_lookup'  InternalRulePriority=Speed  RndMeth=Simplest  InputSameDT=on
      settings: InputPortMap=u0,u1
  Cx : Outport
  Cy : Outport  Port=2
  Cz : Outport  Port=3
  Cl : Outport  Port=4
  Cm : Outport  Port=5
  Cn : Outport  Port=6
  wires:
  [ruddeg] -> Gain5/1
  Cyr lookup/1 -> [Cyr]
  [elevdeg] -> Scope/1, Cm_lookup/2(elev (deg.))
  Demux/11 -> Mux/2
  Demux/9 -> [r]
  [betadeg] -> Cl_lookup/2(beta (deg.))
  [alphadeg] -> Cxq lookup/1, Cyr lookup/1, Cyp lookup/1, Czq lookup/1, Clp lookup5/1, Cnp lookup/1, Cnr lookup/1, Cmq lookup/1, Clr lookup/1
  Product11/1 -> Add7/2
  Demux/8 -> [q]
  Cxq lookup/1 -> [Cxq]
  [Czq] -> Product5/1
  Demux/6 -> Terminator3/1
  Gain3/1 -> [Cq]
  Cmq lookup/1 -> [Cmq]
  Clp lookup5/1 -> [Clp]
  Product16/1 -> Add9/1
  [p] -> Product3/2
  Add2/1 -> Cy/1, [Cy], Display1/1
  Cnr lookup/1 -> [Cnr]
  [betadeg] -> Cn_lookup/2(beta (deg.))
  [alphadeg] -> Cm_lookup/1(alpha (deg.))
  [alphadeg] -> dndr lookup/1, dnda lookup/1, dldr lookup/1, dlda lookup/1
  [Cyr] -> Product4/1
  Cnp lookup/1 -> [Cnp]
  [B2V] -> Product13/1
  Cyp lookup/1 -> [Cyp]
  Czq lookup/1 -> [Czq]
  Clr lookup/1 -> [Clr]
  Add7/1 -> Cm/1
  [r] -> Product4/2
  [Cmq] -> Product11/2
  Gain5/1 -> Product10/2
  Add9/1 -> Product13/2
  [alphadeg] -> Cl_lookup/1(alpha (deg.))
  Demux/5 -> Terminator2/1
  Product4/1 -> Add1/1
  [betadeg] -> Cz_lookup/2(beta (deg.))
  Add8/1 -> Cn/1, Display5/1
  Add1/1 -> Product2/2
  Gain/1 -> [alphadeg]
  Demux/2 -> Gain/1
  [Cq] -> Product5/2
  [aildeg] -> Gain4/1
  [alphadeg] -> Cx_lookup/1(alpha (deg.))
  Add5/1 -> Cl/1, Display3/1
  Cx_lookup/1(Cx) -> Add/1
  Constant1/1 -> Subtract/1
  [Cq] -> Product11/1
  Product5/1 -> Add3/2
  [Cq] -> Product/1
  [dldr] -> Product10/1
  Demux/3 -> Gain1/1
  [alphadeg] -> Cn_lookup/1(alpha (deg.))
  [Cyp] -> Product3/1
  [alphadeg] -> Cz_lookup/1(alpha (deg.))
  Product2/1 -> Add2/2
  dldr lookup/1 -> [dldr]
  [q] -> Product1/2
  Gain6/1 -> Add8/3
  Add3/1 -> Cz/1, [Cz], Display2/1
  Product3/1 -> Add1/2
  control/1 -> Demux1/1
  [dlda] -> Product9/1
  Product18/1 -> Add10/1
  Gain1/1 -> [betadeg]
  [Cnp] -> Product15/1
  [r] -> Product16/2
  [Clr] -> Product8/1
  Product15/1 -> Add9/2
  [p] -> Product15/2
  [Cnr] -> Product16/1
  [aildeg] -> Gain7/1
  [B2V] -> Product6/1
  Divide/1 -> Product1/1, Gain2/1
  [Vt] -> Divide/2
  Add/1 -> Cx/1, Display/1
  Product13/1 -> Add8/2
  [betadeg] -> dlda lookup/2, dldr lookup/2, dnda lookup/2, dndr lookup/2
  Demux/10 -> Mux/1
  Mux/1 -> Terminator/1
  Demux/12 -> Mux/3
  [B2V] -> Product2/1
  Product9/1 -> Add6/1
  Demux1/1 -> Terminator4/1
  Demux1/2 -> [elevdeg]
  Demux1/4 -> [ruddeg]
  Demux1/3 -> [aildeg]
  Product14/1 -> Gain6/1
  [Cz] -> Product12/1
  Add6/1 -> Add5/3
  [Clp] -> Product7/1
  Cz_lookup/1(Cz) -> Add3/1
  Constant2/1 -> Subtract/2
  Gain4/1 -> Product9/2
  [ruddeg] -> Gain8/1
  Add10/1 -> Add8/4
  [Cxq] -> Product/2
  [dnda] -> Product18/1
  Gain7/1 -> Product18/2
  [ruddeg] -> Cy_lookup/3(rudder (deg.))
  [dndr] -> Product17/1
  Constant/1 -> Divide/1
  Gain8/1 -> Product17/2
  Product17/1 -> Add10/2
  [aildeg] -> Cy_lookup/2(aileron (deg.))
  Demux/7 -> [p]
  state/1 -> Demux/1
  [p] -> Product7/2
  Product6/1 -> Add5/2
  Cy_lookup/1(Cy) -> Add2/1
  Product7/1 -> Add4/2
  Demux/1 -> [Vt]
  Demux/4 -> Terminator1/1
  Product1/1 -> Gain3/1
  [elevdeg] -> Cx_lookup/2(elev (deg.))
  Add4/1 -> Product6/2
  Cl_lookup/1(Cl) -> Add5/1
  [elevdeg] -> Cz_lookup/3(elev (deg.))
  [Cy] -> Product14/1
  dnda lookup/1 -> [dnda]
  Product12/1 -> Add7/3
  Gain2/1 -> [B2V]
  Product/1 -> Add/2
  dndr lookup/1 -> [dndr]
  Subtract/1 -> Product12/2
  Demux/13 -> Mux/4
  [r] -> Product8/2
  Cm_lookup/1(Cm) -> Add7/1
  Cn_lookup/1(Cn) -> Add8/1
  dlda lookup/1 -> [dlda]
  Product8/1 -> Add4/1
  [betadeg] -> Cy_lookup/1(beta (deg.))
  Product10/1 -> Add6/2
  Subtract1/1 -> Product14/2
  Constant4/1 -> Subtract1/2
  Constant3/1 -> Subtract1/1

== system f16_simulink/System Dynamics/Power rate of change ==
  state : Inport
  cpow : Inport  Port=2
  Demux : Demux  Outputs=13
  MATLAB Function : MATLAB Function  TreatAsAtomicUnit=on
  Mux : Mux  Inputs=12
  Terminator : Terminator
  Pdot : Outport
  wires:
  MATLAB Function/1(Pdot) -> Pdot/1
  Demux/10 -> Mux/10
  cpow/1 -> MATLAB Function/2(P1)
  Demux/4 -> Mux/4
  Demux/12 -> Mux/12
  Demux/13 -> MATLAB Function/1(P3)
  Demux/2 -> Mux/2
  Demux/11 -> Mux/11
  Demux/1 -> Mux/1
  state/1 -> Demux/1
  Demux/3 -> Mux/3
  Demux/7 -> Mux/7
  Demux/8 -> Mux/8
  Demux/5 -> Mux/5
  Demux/9 -> Mux/9
  Mux/1 -> Terminator/1
  Demux/6 -> Mux/6

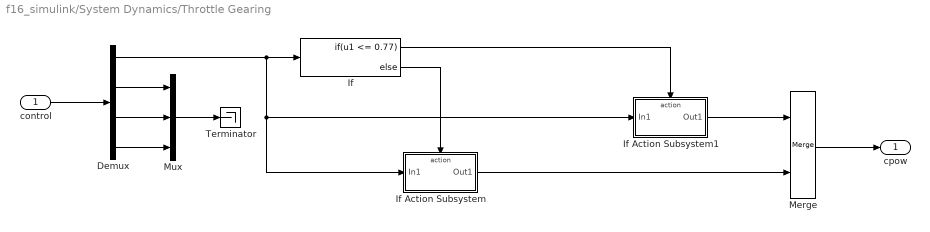
== system f16_simulink/System Dynamics/Throttle Gearing ==
  control : Inport
  Demux : Demux
  If : If  IfExpression=u1 <= 0.77
  If Action Subsystem : Subsystem  TreatAsAtomicUnit=on
  If Action Subsystem1 : Subsystem  TreatAsAtomicUnit=on
  Merge : Merge
  Mux : Mux  Inputs=3
  Terminator : Terminator
  cpow : Outport
  wires:
  If/1 -> If Action Subsystem1/Action
  Mux/1 -> Terminator/1
  control/1 -> Demux/1
  If Action Subsystem/1(Out1) -> Merge/2
  Demux/1 -> If Action Subsystem1/1(In1), If Action Subsystem/1(In1), If/1
  Merge/1 -> cpow/1
  If/2 -> If Action Subsystem/Action
  Demux/3 -> Mux/2
  Demux/2 -> Mux/1
  If Action Subsystem1/1(Out1) -> Merge/1
  Demux/4 -> Mux/3

== system f16_simulink/System Dynamics/Thrust Model ==
  state : Inport
  Demux : Demux  Outputs=13
  Mux : Mux  Inputs=11
  Terminator : Terminator
  n-D Lookup Table : Lookup_n-D  NumberOfTableDimensions=3  BreakpointsForDimension1=altitude_vec  BreakpointsForDimension2=Mach_vec  BreakpointsForDimension3=pow_vec  Table=power_table  ExtrapMethod=Clip  InternalRulePriority=Speed  RndMeth=Simplest  InputSameDT=on
      settings: InputPortMap=u0,u1,u2
  thrust : Outport
  wires:
  [M] -> n-D Lookup Table/2
  Mux/1 -> Terminator/1
  Demux/13 -> n-D Lookup Table/3  "power"
  Demux/6 -> Mux/6
  state/1 -> Demux/1
  Demux/11 -> Mux/11
  Demux/9 -> Mux/9
  Demux/3 -> Mux/3
  Demux/12 -> n-D Lookup Table/1  "altitude"
  Demux/7 -> Mux/7
  n-D Lookup Table/1 -> thrust/1
  Demux/2 -> Mux/2
  Demux/1 -> Mux/1
  Demux/5 -> Mux/5
  Demux/8 -> Mux/8
  Demux/10 -> Mux/10
  Demux/4 -> Mux/4

== system f16_simulink/Theta Square Wave Generator/If Action Subsystem ==
  In1 : Inport
  Action Port : ActionPort  ActionPortLabel=else
  Out1 : Outport
  wires:
  In1/1 -> Out1/1

== system f16_simulink/Theta Square Wave Generator/If Action Subsystem2 ==
  In1 : Inport
  Action Port : ActionPort  ActionPortLabel=if(u1 > wavestart)
  Constant : Constant  Value=thetaref_amp
  Subtract : Sum  Inputs=+-
  Out1 : Outport
  wires:
  Constant/1 -> Subtract/2
  Subtract/1 -> Out1/1
  In1/1 -> Subtract/1

== system f16_simulink/System Dynamics/ADC/If Action Subsystem ==
  In1 : Inport
  Action Port : ActionPort  ActionPortLabel=else
  Out1 : Outport
  wires:
  In1/1 -> Out1/1

== system f16_simulink/System Dynamics/ADC/If Action Subsystem1 ==
  In1 : Inport
  Action Port : ActionPort  ActionPortLabel=if(u1 > 35000)
  Out1 : Outport
  wires:
  In1/1 -> Out1/1

== system f16_simulink/System Dynamics/Aerodynamic Model/Cl_lookup ==
  alpha (deg.) : Inport
  beta (deg.) : Inport  Port=2
  Abs : Abs
  Cl_table : Lookup_n-D  BreakpointsForDimension1=alpha_vec  BreakpointsForDimension2=beta_vec5  BreakpointsForDimension3=[5, 7]  Table=Cl_lookup'  InternalRulePriority=Speed  RndMeth=Simplest  InputSameDT=on
      settings: InputPortMap=u0,u1
  Product : Product
  Sign : Signum
  Cl : Outport
  wires:
  Cl_table/1 -> Product/1
  Product/1 -> Cl/1
  beta (deg.)/1 -> Sign/1, Abs/1
  alpha (deg.)/1 -> Cl_table/1
  Abs/1 -> Cl_table/2
  Sign/1 -> Product/2

== system f16_simulink/System Dynamics/Aerodynamic Model/Cm_lookup ==
  alpha (deg.) : Inport
  elev (deg.) : Inport  Port=2
  Cm_table : Lookup_n-D  BreakpointsForDimension1=alpha_vec  BreakpointsForDimension2=elev_vec  BreakpointsForDimension3=[5, 7]  Table=Cm_lookup'  InternalRulePriority=Speed  RndMeth=Simplest  InputSameDT=on
      settings: InputPortMap=u0,u1
  Cm : Outport
  wires:
  elev (deg.)/1 -> Cm_table/2
  Cm_table/1 -> Cm/1
  alpha (deg.)/1 -> Cm_table/1

== system f16_simulink/System Dynamics/Aerodynamic Model/Cn_lookup ==
  alpha (deg.) : Inport
  beta (deg.) : Inport  Port=2
  Abs : Abs
  Cn_table : Lookup_n-D  BreakpointsForDimension1=alpha_vec  BreakpointsForDimension2=beta_vec5  BreakpointsForDimension3=[5, 7]  Table=Cn_lookup'  InternalRulePriority=Speed  RndMeth=Simplest  InputSameDT=on
      settings: InputPortMap=u0,u1
  Product : Product
  Sign : Signum
  Cn : Outport
  wires:
  Cn_table/1 -> Product/1
  Product/1 -> Cn/1
  alpha (deg.)/1 -> Cn_table/1
  beta (deg.)/1 -> Sign/1, Abs/1
  Sign/1 -> Product/2
  Abs/1 -> Cn_table/2

== system f16_simulink/System Dynamics/Aerodynamic Model/Cx_lookup ==
  alpha (deg.) : Inport
  elev (deg.) : Inport  Port=2
  Cx_table : Lookup_n-D  BreakpointsForDimension1=alpha_vec  BreakpointsForDimension2=elev_vec  BreakpointsForDimension3=[5, 7]  Table=Cx_lookup'  InternalRulePriority=Speed  RndMeth=Simplest  InputSameDT=on
      settings: InputPortMap=u0,u1
  Cx : Outport
  wires:
  Cx_table/1 -> Cx/1
  elev (deg.)/1 -> Cx_table/2
  alpha (deg.)/1 -> Cx_table/1

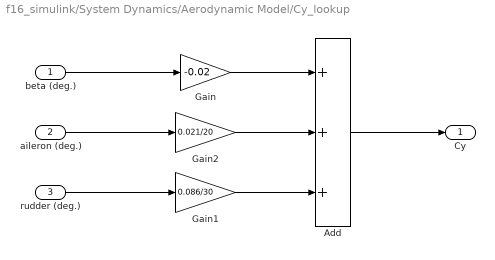
== system f16_simulink/System Dynamics/Aerodynamic Model/Cy_lookup ==
  beta (deg.) : Inport
  aileron (deg.) : Inport  Port=2
  rudder (deg.) : Inport  Port=3
  Add : Sum  Inputs=+++
  Gain : Gain  Gain=-0.02
  Gain1 : Gain  Gain=0.086/30
  Gain2 : Gain  Gain=0.021/20
  Cy : Outport
  wires:
  aileron (deg.)/1 -> Gain2/1
  rudder (deg.)/1 -> Gain1/1
  Add/1 -> Cy/1
  Gain/1 -> Add/1
  Gain2/1 -> Add/2
  Gain1/1 -> Add/3
  beta (deg.)/1 -> Gain/1

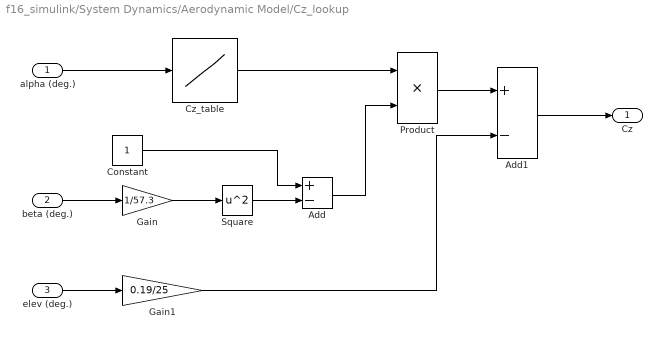
== system f16_simulink/System Dynamics/Aerodynamic Model/Cz_lookup ==
  alpha (deg.) : Inport
  beta (deg.) : Inport  Port=2
  elev (deg.) : Inport  Port=3
  Add : Sum  Inputs=+-
  Add1 : Sum  Inputs=+-
  Constant : Constant
  Cz_table : Lookup_n-D  NumberOfTableDimensions=1  BreakpointsForDimension1=alpha_vec  Table=Cz_lookup  InternalRulePriority=Speed  RndMeth=Simplest  InputSameDT=on
  Gain : Gain  Gain=1/57.3
  Gain1 : Gain  Gain=0.19/25
  Product : Product
  Square : Math  Operator=square  SaturateOnIntegerOverflow=on
  Cz : Outport
  wires:
  Constant/1 -> Add/1
  Add1/1 -> Cz/1
  Add/1 -> Product/2
  alpha (deg.)/1 -> Cz_table/1
  Gain1/1 -> Add1/2
  Gain/1 -> Square/1
  Cz_table/1 -> Product/1
  elev (deg.)/1 -> Gain1/1
  beta (deg.)/1 -> Gain/1
  Square/1 -> Add/2
  Product/1 -> Add1/1

== system f16_simulink/System Dynamics/Throttle Gearing/If Action Subsystem ==
  In1 : Inport
  Action Port : ActionPort  ActionPortLabel=else
  Constant : Constant  Value=117.38
  Gain : Gain  Gain=217.38
  Subtract : Sum  Inputs=+-
  Out1 : Outport
  wires:
  In1/1 -> Gain/1
  Subtract/1 -> Out1/1
  Gain/1 -> Subtract/1
  Constant/1 -> Subtract/2

== system f16_simulink/System Dynamics/Throttle Gearing/If Action Subsystem1 ==
  In1 : Inport
  Action Port : ActionPort  ActionPortLabel=if(u1 <= 0.77)
  Gain : Gain  Gain=64.94
  Out1 : Outport
  wires:
  In1/1 -> Gain/1
  Gain/1 -> Out1/1

== matlab function f16_simulink/System Dynamics/Power rate of change/MATLAB Function ==
  data: P3 input; Pdot output; P1 input
function Pdot = f16_Pdot(P3,P1)
    % P3: actual power
    % P1: power command
    
    if P1 >= 50
        if P3 >= 50
            T = 5;
            P2 = P1;
        else
            P2 = 60;
            T = f16_Rtau(P2-P3);
        end
    else
        if P3 >= 50
            T = 5;
            P2 = 40;
        else
            P2 = P1;
            T = f16_Rtau(P2-P3);
        end
    end
    
    Pdot = T*(P2-P3);

end

function Rtau = f16_Rtau(dP)
    % reciprocal time constant
    if dP <= 25
        Rtau  = 1;
    elseif dP >= 50
        Rtau = 0.1;
    else
        Rtau = 1.9 - 0.036*dP;
    end
end
